simulink model "PIcranesimu"  (R2015a)
settings: Solver=ode45  StartTime=0.0  StopTime=20  RelTol=1e-3
libraries: cstblocks x3, simulink x1
settings Model: Creator=roevhat  LastModifiedBy=Steffan

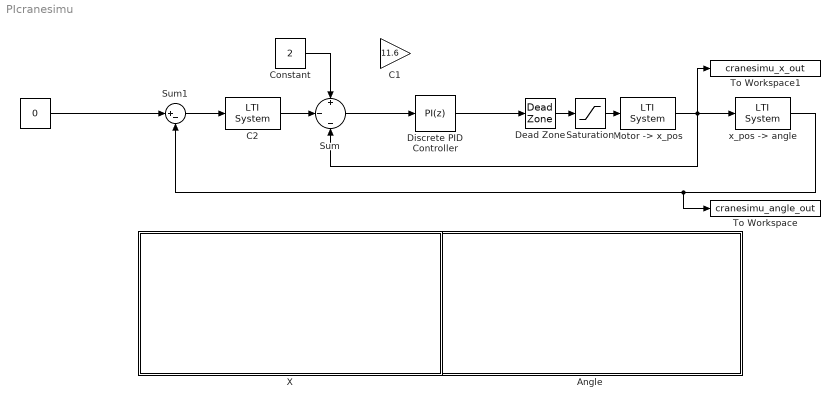
== system PIcranesimu ==
  " " : Constant  Value=0
  Angle : Subsystem  DialogController=hmiCreateDDGDialog  IsWebBlock=on  mask(MathWorksWebBlock){webBlockId=a8e75964-e3a8-414a-b4cf-d80626da48bf, webBlockType=sdiscope, ShowInitialText=on, HMISrcModelName=cranesimu}
      mask prompts: webBlockId "WebBlock Id"; webBlockType "WebBlock Type"; HMISrcModelName "Source Model"
      mask Help: helpview([docroot '/mapfiles/simulink.map'], 'hmi_scope')
      mask Display:
      | if strcmp(get_param(bdroot(gcb),'BlockDiagramType'), 'library')
      |     image([(matlabroot) '/toolbox/simulink/hmi/icons/DashboardScope.png']);
      | end
  C1 : Gain  Gain=11.6
  C2 : cstblocks/LTI System  sys=C2  IC=[]
  Constant : Constant  Value=2
  Dead Zone : DeadZone  LowerValue=-5  UpperValue=5  SaturateOnIntegerOverflow=on
  Discrete PID Controller : simulink/Continuous/PID Controller  Controller=PI  TimeDomain=Discrete-time  SampleTime=0.02  IntegratorMethod=Forward Euler  FilterMethod=Forward Euler  Form=Parallel  UseFilter=on  ControllerParametersSource=internal  P=11.6  I=4.5  D=0.303969850834222  N=32.571148723477  InitialConditionSource=internal  InitialConditionForIntegrator=0  InitialConditionForFilter=0  ExternalReset=none  LimitOutput=off  UpperSaturationLimit=inf  LowerSaturationLimit=-inf  LinearizeAsGain=off  AntiWindupMode=none  Kb=1  TrackingMode=off  Kt=1  PParamMin=[]  PParamMax=[]  IParamMin=[]  IParamMax=[]  DParamMin=[]  DParamMax=[]  NParamMin=[]  NParamMax=[]  KbParamMin=[]  KbParamMax=[]  KtParamMin=[]  KtParamMax=[]  POutMin=[]  POutMax=[]  IOutMin=[]  IOutMax=[]  DOutMin=[]  DOutMax=[]  NOutMin=[]  NOutMax=[]  KbOutMin=[]  KbOutMax=[]  KtOutMin=[]  KtOutMax=[]  IntegratorOutMin=[]  IntegratorOutMax=[]  FilterOutMin=[]  FilterOutMax=[]  SumOutMin=[]  SumOutMax=[]  SumI1OutMin=[]  SumI1OutMax=[]  SumI2OutMin=[]  SumI2OutMax=[]  SumI3OutMin=[]  SumI3OutMax=[]  SumDOutMin=[]  SumDOutMax=[]  SaturationOutMin=[]  SaturationOutMax=[]  IntegratorContinuousStateAttributes=''  IntegratorStateMustResolveToSignalObject=off  IntegratorRTWStateStorageClass=Auto  FilterContinuousStateAttributes=''  FilterStateMustResolveToSignalObject=off  FilterRTWStateStorageClass=Auto  DifferentiatorICPrevScaledInput=0  DifferentiatorOutMin=[]  DifferentiatorOutMax=[]
  "Motor -> x_pos" : cstblocks/LTI System  sys=X  IC=[]
  Saturation : Saturate  UpperLimit=14  LowerLimit=-14
  Sum : Sum  Inputs=+|-|-
  Sum1 : Sum  Inputs=|+-
  To Workspace : ToWorkspace  VariableName=cranesimu_angle_out  SaveFormat=Timeseries  SampleTime=-1
  To Workspace1 : ToWorkspace  VariableName=cranesimu_x_out  SaveFormat=Timeseries  SampleTime=-1
  X : Subsystem  DialogController=hmiCreateDDGDialog  IsWebBlock=on  mask(MathWorksWebBlock){webBlockId=2ac42065-2a1d-45d8-b9d1-76f78bc34ac1, webBlockType=sdiscope, ShowInitialText=on, HMISrcModelName=cranesimu}
      mask prompts: webBlockId "WebBlock Id"; webBlockType "WebBlock Type"; HMISrcModelName "Source Model"
      mask Help: helpview([docroot '/mapfiles/simulink.map'], 'hmi_scope')
      mask Display:
      | if strcmp(get_param(bdroot(gcb),'BlockDiagramType'), 'library')
      |     image([(matlabroot) '/toolbox/simulink/hmi/icons/DashboardScope.png']);
      | end
  "x_pos -> angle" : cstblocks/LTI System  sys=W  IC=[]
  wires:
  "Motor -> x_pos"/1 -> To Workspace1/1, "x_pos -> angle"/1, Sum/3
  "x_pos -> angle"/1 -> To Workspace/1, Sum1/2
  " "/1 -> Sum1/1
  Sum1/1 -> C2/1
  Saturation/1 -> "Motor -> x_pos"/1
  C2/1 -> Sum/2
  Dead Zone/1 -> Saturation/1
  Constant/1 -> Sum/1
  Discrete PID Controller/1 -> Dead Zone/1
  Sum/1 -> Discrete PID Controller/1

== system PIcranesimu/Angle ==

== system PIcranesimu/X ==
